simulink model "fir"  (R2025a)
settings: Solver=VariableStepAuto  StartTime=0.0  StopTime=4096*1/200e6  RelTol=1e-3
InitFcn:
  | set_params
model workspace (MAT data in the model file):
  cascade_stage = 6
  frame_size = 1024
  max_fft_size = 1024
  window_size = 256
undefined symbols (not defined in the file or in its folder): None, S, vsva2197, xcvc1902, xlfda_numerator
libraries: aieBasic x2, aieDSP x1, simulink x1, hdlUtilities x1, vmcUtilities x1, dspobslib x1, aieUtilities x1
settings Model: Creator=abehbood  LastModifiedBy=sdegala
settings SolverCC: AlgebraicLoopSolver=TrustRegion
settings DebuggingCC: UnconnectedInputMsg=warning  UnconnectedOutputMsg=warning  UnconnectedLineMsg=warning
settings ModelReferenceCC: EnableRefExpFcnMdlSchedulingChecks=on
settings RTWCC: GPUComputeCapability=3.5  DLArmComputeVersion=19.05

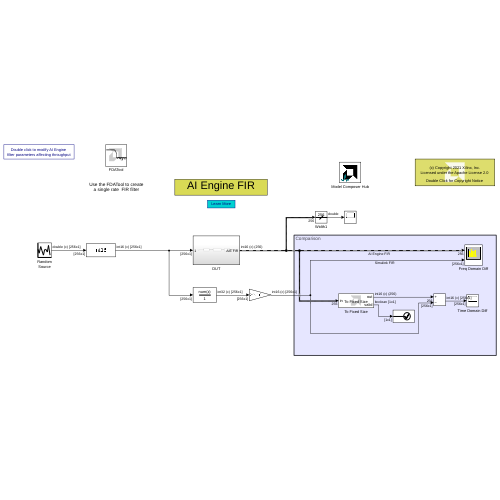
[thumbnail: Simulink's stored preview of the top-level diagram]
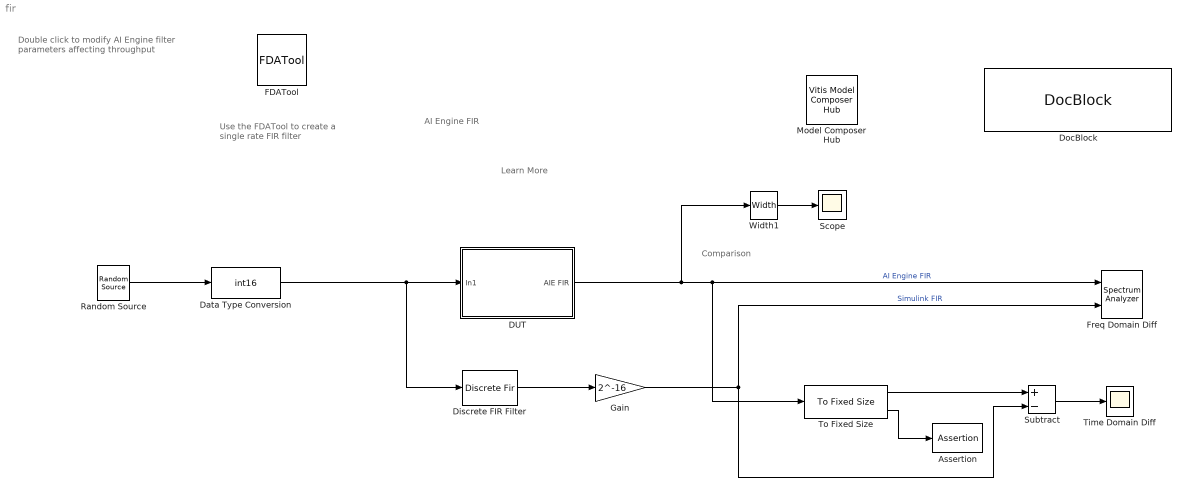
== system fir ==
  note: Double click to modify AI Engine
      | filter parameters affecting throughput
  note: Learn More
  note: Comparison
  note: Use the FDATool to create
      | a single rate FIR filter
  note: AI Engine FIR
  Assertion : Assertion
  DUT : Subsystem
  Data Type Conversion : DataTypeConversion  OutDataTypeStr=int16  SaturateOnIntegerOverflow=off  RndMeth=Floor
  Discrete FIR Filter : DiscreteFir  Coefficients=int16(xlfda_numerator(strcat(bdroot,'/FDATool'))*2^15)  InputProcessing=Columns as channels (frame based)  CoefDataTypeStr=int16  ProductDataTypeStr=fixdt(1,32,0)  AccumDataTypeStr=fixdt(1,48,0)  OutDataTypeStr=fixdt(1,32,0)  SaturateOnIntegerOverflow=on
  DocBlock : simulink/Model-Wide Utilities/DocBlock  DocumentType=Text  mask(DocBlock){}
      content=|
      | ///////////////////////////////////////////////////////////////////////////
      | // Copyright 2020 Xilinx
      | //
      | // Licensed under the Apache License, Version 2.0 (the "License");
      | // you may not use this file except in compliance with the License.
      | // You may obtain a copy of the License at
      | //
      | // http://www.apache.org/licenses/LICENSE-2.0
      | //
      | // Unless required by applicable law or agreed to in writing, software
      | // distributed under the License is distributed on an "AS IS" BASIS,
      | // WITHOUT WARRANTIES OR CONDITIONS OF ANY KIND, either express or implied.
      | // See the License for the specific language governing permissions and
      | // limitations under the License.
      | ///////////////////////////////////////////////////////////////////////////
      mask Display:
      | xmcDrawBlockIcon();
      | disp(['{\fontsize{10pt}(c) Copyright 2021' ' Xilinx, Inc.}\newline \newline '],'texmode','on');
      | disp('{\fontsize{10pt}Licensed under the Apache License 2.0}','texmode','on');
      | disp('\newline \newline \newline{\fontsize{10pt}Double Click for Copyright Notice}','texmode','on');
  FDATool : hdlUtilities/FDATool  block_type=fdatool
      settings: infoedit=FDATool
  Freq Domain Diff : SpectrumAnalyzer  NumInputPorts=2  WindowPosition=[322.000000,188.000000,882.000000,415.000000,]  ScopeFrameLocation=window  Method=Welch  SampleRate=200000000  Span=200000000  StartFrequency=-100000000  StopFrequency=100000000  AveragingMethod=Exponential  YLimits=[6.3733 98.9865]  ShowLegend=on  ChannelNames="[\"\"]"  AllowFFTLengthLessThanSamplesPerUpdate=on  DefaultConfigurationName=spbscopes.SpectrumAnalyzerBlockCfg
  Gain : Gain  Gain=2^-16  OutDataTypeStr=int16
  Model Composer Hub : vmcUtilities/Vitis Model Composer Hub  Tag=genX  CodeGeneration=off  SubsystemName=DUT  BlockHierPath=fir/DUT  SubsystemType=AIENode  AIEArrayConfig=Use entire AIE array  StartColumn=1  NumberOfColumns=1  TargetDirectory=./code  exportDesign=on  analyzeDesign=off  validateDesignOnHw=off  ExportType=AI Engines  IpVendor=xilinx.com  IpLibrary=hls  IpVersion=1.0  IpHWLanguage=Verilog  AieCompilerOptions={}  AieSimulatorOptions={}  CreateTestbench=on  TestbenchStackSize=10  RunRtlSim=off  RunCSim=off  RunAieSim=on  AieSimTimeout=50000  RunAieSimProfiling=off  LaunchVitisAnalyzer=off  PlotOutput=on  RunX86Sim=off  X86SimTimeout=10  GenHwImage=off  GenLibadfXo=off  GenHwValidationCode=off  PlatformType=Specify Platform  Platform=/proj/xbuilds/SWIP/9999.0_0721_1752/installs/lin64/2025.2/Vitis/base_platforms/xilinx_vck190_base_202520_1/xilinx_vck190_base_202520_1.xpfm  HwSystemType=Baremetal  HwValidationTarget=hw  ProjDevice=Versal VCK190 Evaluation Platform (xcvc1902-vsva2197-2MP-e-S)  ProjDevicePart=xcvc1902-vsva2197-2MP-e-S  AIEType=AIE  SamplePeriod=-1  ClockFrequency=200  DataPathParallelism=1  xilinxfamily=versalaicore  part=xcvc1902  speed=-2MP-e-S  package=vsva2197  directory=./netlist  testbench=off  incr_netlist=off  synthesis_tool=Vivado  clock_wrapper=Clock Enables  dbl_ovrd=According to Block Masks  dcm_input_clock_period=10  sysclk_period=10  simulink_period=1  eval_field=0  IPInfoJsonString="{\"DUTSubsystemName\":\"DUT\",\"AIESubsystem\":{\"SubsystemName\":\"DUT\",\"TargetDirectory\":\"./code\",\"AIEArrayConfig\":\"Use entire AIE array\",\"StartColumn\":\"0\",\"NumberOfColumns\":\"1\"},\"SubsystemTag\":\"AIENode\"}"  LogFileName=/proj/xhdhdstaff5/sdegala/Head1/HEAD/VMC_JULY_LATEST/Vitis_Model_Composer/Examples/AIENGINE/DSPlib/fir/code/model_composer.log  NThreads=4  IPConfigFile=/tmp/vmctmp-9387929265040231051/fir_ipconfig.json
  Random Source : dspobslib/Random Source  SrcType=Uniform  NormMethod=Sum of uniform values  CltLength=12  MinVal=-2^15  MaxVal=2^15-1  MeanVal=0  VarVal=50  RepMode=Not repeatable  rawSeed=1  IsInherit=off  SampMode=Discrete  SampTime=1/200e6  SampFrame=window_size  DataType=Double  OutComplex=Complex  OutputFrames=off
  Scope : Scope
      settings: ActiveDisplayYMinimum=156  ActiveDisplayYMaximum=356
  Subtract : Sum  Inputs=+-
  Time Domain Diff : Scope
      settings: ActiveDisplayYMinimum=-1  ActiveDisplayYMaximum=1
  To Fixed Size : aieUtilities/To Fixed Size  Mode=Produce a valid output signal  OutputSize=Inherit: Same as input  CopyMethod=Buffer samples to form output  HasStatusOutput=on
  Width1 : Width
  wires:
  Width1/1 -> Scope/1
  Discrete FIR Filter/1 -> Gain/1
  Data Type Conversion/1 -> Discrete FIR Filter/1, DUT/1(In1)
  To Fixed Size/1 -> Subtract/1
  To Fixed Size/2 -> Assertion/1
  Subtract/1 -> Time Domain Diff/1
  Random Source/1 -> Data Type Conversion/1
  DUT/1(AIE FIR) -> Width1/1, To Fixed Size/1, Freq Domain Diff/1  "AI Engine FIR"
  Gain/1 -> Freq Domain Diff/2, Subtract/2  "Simulink FIR"

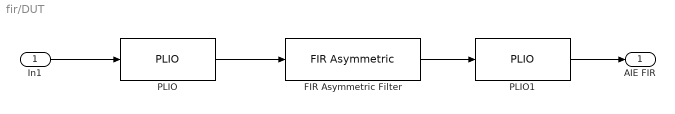
== system fir/DUT ==
  In1 : Inport
  FIR Asymmetric Filter : aieDSP/FIR Asymmetric  data_type=cint16  coef_type=cint16  use_coeff_reload=off  num_outputs=off  coeff=int16(xlfda_numerator(strcat(bdroot,'/FDATool'))*2^15)  fir_length=32  input_window_size=window_size  shift_val=16  rnd_mode=Floor  sat_mode=0-None  casc_length=cascade_stage  AIE_VARIANT=1  TP_API=0  dual_ip=0  ssr=1  blockJsonConstraints=[]  blockJsonConstraintsInternal=[]  spec=vmc_fir_sr_asym.json  SerializedMaskParamNames=[]  SerializedMaskParamValues=[]  SerializedMaskParamVisibilities=[]  block_type=FIR Asymmetric  SerializedMaskParamDataypes=typename|typename|uint|uint|coef_type|uint|uint|uint|uint|uint|uint|uint|uint|uint|uint  SerializedMaskParamEnumStrArr=0|0|0|0|0|0|0|0|Floor,Ceiling,Round to positive infinity,Round to negative infinity,Round symmetrical to infinity,Round symmetrical to zero,Round convergent to even,Round convergent to odd|0-None,1-Asymmetric,3-Symmetric|0|0|0|0|0  SerializedMaskParamEnumValArr=0|0|0|0|0|0|0|0|0,1,2,3,4,5,6,7|0,1,3|0|0|0|0|0  SerializedMaskParamVectorArr=0|0|0|0|1|0|0|0|0|0|0|0|0|0|0  SerializedMaskParamKeys=TT_DATA|TT_COEFF|TP_USE_COEFF_RELOAD|TP_NUM_OUTPUTS|coeff|TP_FIR_LEN|TP_INPUT_WINDOW_VSIZE|TP_SHIFT|TP_RND|TP_SAT|TP_CASC_LEN|AIE_VARIANT|TP_API|TP_DUAL_IP|TP_SSR
  PLIO : aieBasic/PLIO  PlioWidth=64  PlioFreqSpec=on  PlioFreq=500  ColLocation=0  channel=0  blockJsonConstraints=[]  deprecateConstraints=0
  PLIO1 : aieBasic/PLIO  PlioWidth=64  PlioFreqSpec=on  PlioFreq=500  ColLocation=0  channel=0  blockJsonConstraints=[]  deprecateConstraints=0
  AIE FIR : Outport
  wires:
  In1/1 -> PLIO/1
  FIR Asymmetric Filter/1 -> PLIO1/1
  PLIO/1 -> FIR Asymmetric Filter/1
  PLIO1/1 -> AIE FIR/1
